simulink model "tank_with_compressibility"  (R2025b)
settings: Solver=VariableStepAuto  StartTime=0.0  StopTime=10.0  RelTol=1e-3
model workspace (MAT data in the model file):
  P0 = Simulink.Parameter
  P0.Value = 300
  P0.Complexity = 'real'
  P0.Dimensions = [1 1]
  P0.DataType = 'auto'
  T0 = Simulink.Parameter
  T0.Value = 40.5939137189
  T0.Complexity = 'real'
  T0.Dimensions = [1 1]
  T0.DataType = 'auto'
  mdotGain = Simulink.Parameter
  mdotGain.Value = 1.32504710711e-08
  mdotGain.Complexity = 'real'
  mdotGain.Dimensions = [1 1]
  mdotGain.DataType = 'auto'
undefined symbols (not defined in the file): Cv, Patm, R, V
settings Model: Creator=karadeli  LastModifiedBy=karadeli

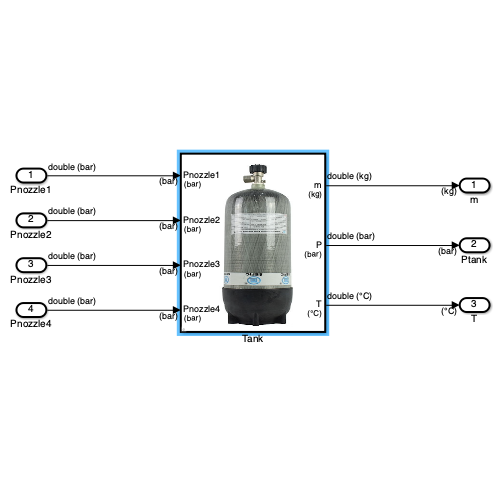
[thumbnail: Simulink's stored preview of the top-level diagram]
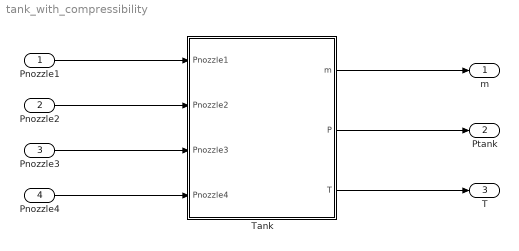
== system tank_with_compressibility ==
  Pnozzle1 : Inport
  Pnozzle2 : Inport  Port=2
  Pnozzle3 : Inport  Port=3
  Pnozzle4 : Inport  Port=4
  Tank : Subsystem  mask{P0=300, T0=40.5939, mdotGain=mdotGain}
      mask Display: image('Tank.png');
  m : Outport  Unit=kg
  Ptank : Outport  Port=2  Unit=bar
  T : Outport  Port=3  Unit=°C
  wires:
  Pnozzle1/1 -> Tank/1(Pnozzle1)
  Tank/1(m) -> m/1
  Tank/2(P) -> Ptank/1
  Pnozzle2/1 -> Tank/2(Pnozzle2)
  Pnozzle3/1 -> Tank/3(Pnozzle3)
  Pnozzle4/1 -> Tank/4(Pnozzle4)
  Tank/3(T) -> T/1

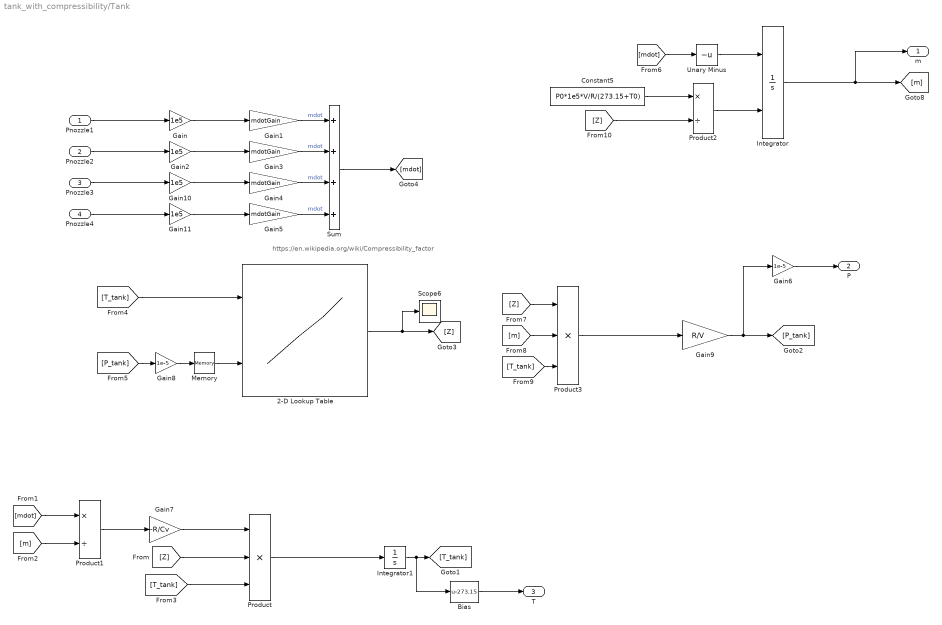
== system tank_with_compressibility/Tank ==
  note: https://en.wikipedia.org/wiki/Compressibility_factor
  Pnozzle1 : Inport  Unit=bar
  Pnozzle2 : Inport  Port=2  Unit=bar
  Pnozzle3 : Inport  Port=3  Unit=bar
  Pnozzle4 : Inport  Port=4  Unit=bar
  2-D Lookup Table : Lookup_n-D  BreakpointsForDimension1=[75;80;90;100;120;140;160;180;200;250;300;350;400;450;500;600;800;1000]  BreakpointsForDimension2=[1;5;10;20;40;60;80;100;150;200;250;300;400;500]  Table=[0.0052 0.0260 0.0519 0.1036 0.2063 0.3082 0.4094 0.5099 0.7581 1.0125 0.0000 0.0000 0.0000 0.0000;0.0000 0.0250 0.0499 0.0995 0.1981 0.2958 0.3927 0.4887 0.7258 0.9588 1.1931 1.4139 0.0000 0.0000;0.9764 0.0236 0.0453 0.0940 0.1866 0.2781 0.3686 0.4681 0.6779 0.8929 1.1098 1.3110 1.7161 2.1105;0.9797 0.8872 0.0453 0.0900 0.1782 0.2635 0.3498 0.4337 0.6386 0.8377 1.0395 1.2227 1.5937 1.9536;0.9880 0.9373 0.8860 0.6730 0.1778 0.2557 0.3371 0.4132 0.5964 0.7720 0.9530 1.1076 1.5091 1.7366;0.9927 0.9614 0.9205 0.8297 0.5856 0.3313 0.3737 0.4340 0.5909 0.7699 0.9114 1.0393 1.3202 1.5903;0.9951 0.9748 0.9489 0.8954 0.7803 0.6603 0.5696 0.5489 0.6340 0.7564 0.8840 1.0105 1.2585 1.4970;0.9967 0.9832 0.9660 0.9314 0.8625 0.7977 0.7432 0.7084 0.7180 0.7986 0.9000 1.0068 1.2232 1.4361;0.9978 0.9886 0.9767 0.9539 0.9100 0.8701 0.8374 0.8142 0.8061 0.8549 0.9311 1.0185 1.2054 1.3944;0.9992 0.9957 0.9911 0.9822 0.9671 0.9549 0.9463 0.9411 0.9450 0.9713 1.0152 1.0702 1.1990 1.3392;0.9999 0.9987 0.9974 0.9950 0.9917 0.9901 0.9903 0.9930 1.0074 1.0326 1.0669 1.1089 1.2073 1.3163;1.0000 1.0002 1.0004 1.0014 1.0038 1.0075 1.0121 1.0183 1.0377 1.0635 1.0947 1.1303 1.2116 1.3015;1.0002 1.0012 1.0025 1.0046 1.0100 1.0159 1.0229 1.0312 1.0533 1.0795 1.1087 1.1411 1.2117 1.2890;1.0003 1.0016 1.0034 1.0063 1.0133 1.0210 1.0287 1.0374 1.0614 1.0913 1.1183 1.1463 1.2090 1.2778;1.0003 1.0020 1.0034 1.0074 1.0151 1.0234 1.0323 1.0410 1.0650 1.0913 1.1183 1.1463 1.2051 1.2667;1.0004 1.0022 1.0039 1.0081 1.0164 1.0253 1.0340 1.0434 1.0678 1.0920 1.1172 1.1427 1.1947 1.2475;1.0004 1.0020 1.0038 1.0077 1.0157 1.0240 1.0321 1.0408 1.0621 1.0844 1.1061 1.1283 1.1720 1.2150;1.0004 1.0018 1.0037 1.0068 1.0142 1.0215 1.0290 1.0365 1.0556 1.0744 1.0948 1.1131 1.1515 1.1889]  InternalRulePriority=Speed  RndMeth=Simplest
      settings: InputPortMap=u0,u1
  Bias : Bias  Bias=-273.15  SaturateOnIntegerOverflow=off
  Constant5 : Constant  Value=P0*1e5*V/R/(273.15+T0)
  Gain{,2,10..11} (4 alike) : Gain  Gain=1e5
  Gain{1,3..5} (4 alike) : Gain  Gain=mdotGain
  Gain6 : Gain  Gain=1e-5
  Gain7 : Gain  Gain=-R/Cv
  Gain8 : Gain  Gain=1e-5
  Gain9 : Gain  Gain=R/V
  Integrator : Integrator  InitialConditionSource=external  InitialCondition=3  LimitOutput=on  UpperSaturationLimit=5  LowerSaturationLimit=Patm*V/R/100
  Integrator1 : Integrator  InitialCondition=T0+273.15  LowerSaturationLimit=0
  Memory : Memory  InitialCondition=P0
  Product : Product  Inputs=3
  Product1 : Product  Inputs=*/
  Product2 : Product  Inputs=*/
  Product3 : Product  Inputs=3
  Scope6 : Scope
      settings: ActiveDisplayYMinimum=0.8767629134747118  ActiveDisplayYMaximum=1.1251537258363551  DataLoggingVariableName=ScopeData19
  Sum : Sum  Inputs=4
  Unary Minus : UnaryMinus
  m : Outport  Unit=kg
  P : Outport  Port=2  Unit=bar
  T : Outport  Port=3  Unit=°C
  wires:
  Gain1/1 -> Sum/1  "mdot"
  Pnozzle1/1 -> Gain/1
  Unary Minus/1 -> Integrator/1
  Integrator/1 -> m/1, [m]
  [mdot] -> Unary Minus/1
  Constant5/1 -> Product2/1
  Pnozzle2/1 -> Gain2/1
  Pnozzle3/1 -> Gain10/1
  Pnozzle4/1 -> Gain11/1
  Gain5/1 -> Sum/4  "mdot"
  Gain4/1 -> Sum/3  "mdot"
  Gain3/1 -> Sum/2  "mdot"
  Sum/1 -> [mdot]
  Bias/1 -> T/1
  Gain6/1 -> P/1
  Gain7/1 -> Product/1
  Product/1 -> Integrator1/1
  Product1/1 -> Gain7/1
  [m] -> Product1/2
  Integrator1/1 -> Bias/1, [T_tank]
  [mdot] -> Product1/1
  [Z] -> Product/2
  [T_tank] -> Product/3
  Gain8/1 -> Memory/1
  2-D Lookup Table/1 -> [Z], Scope6/1
  [T_tank] -> 2-D Lookup Table/1
  [P_tank] -> Gain8/1
  Memory/1 -> 2-D Lookup Table/2
  Product3/1 -> Gain9/1
  Gain9/1 -> Gain6/1, [P_tank]
  [Z] -> Product3/1
  [m] -> Product3/2
  [T_tank] -> Product3/3
  Product2/1 -> Integrator/2
  [Z] -> Product2/2
  Gain/1 -> Gain1/1
  Gain2/1 -> Gain3/1
  Gain10/1 -> Gain4/1
  Gain11/1 -> Gain5/1
